simulink model "MyBatteryCU_RTW"  (Simulink 8.7)
settings: Solver=ode1  SolverMode=SingleTasking  StartTime=0.0  StopTime=inf  FixedStep=0.0002  RelTol=1e-3
PreLoadFcn:
  | vehicle = 'Car'; if ~length(which('cmcmd')), cmenv; end
  | MyBatteryCU_RTW_bus
InitFcn:
  | vehicle = 'Car'; if ~length(which('cmcmd')), cmenv; end
  | MyBatteryCU_RTW_bus
Description:
  | CarMaker Plug-in Model Target
settings Model: Creator=ml  LastModifiedBy=IPG
settings DataIOCC: SignalLoggingSaveFormat=ModelDataLogs
settings OptimizationCC: ExpressionDepthLimit=2147483647
settings DebuggingCC: FcnCallInpInsideContextMsg=UseLocalSettings  StateNameClashWarn=warning
settings HardwareCC: TargetHWDeviceType=32-bit Generic  ProdEqTarget=off
settings RTWCC: SystemTargetFile=CarMaker.tlc  TemplateMakefile=CarMaker_unix-win64.tmf  Description=CarMaker Plug-in Model Target
settings CodeAppCC: MaxIdLength=63
settings STFCustomTargetCC: ModelReferenceCompliant=off  GeneratePreprocessorConditionals=Disable all  MultiInstanceERTCode=on  CodeInterfacePackaging=Reusable function  CPPClassGenCompliant=on  GRTInterface=off  GenerateAllocFcn=on  SystemTargetFile=CarMaker.tlc
settings GRTTargetCC: ModelReferenceCompliant=off  ParMdlRefBuildCompliant=off  CompOptLevelCompliant=off  ConcurrentExecutionCompliant=off  CombineOutputUpdateFcns=off  MatFileLogging=off  MultiInstanceERTCode=on  CodeInterfacePackaging=Reusable function  GenerateAllocFcn=on  UseToolchainInfoCompliant=off  ExtModeMexFile=noextcomm
settings CustomProperty: DataType=string  Value=..
settings EnumStrPairs: String=Car

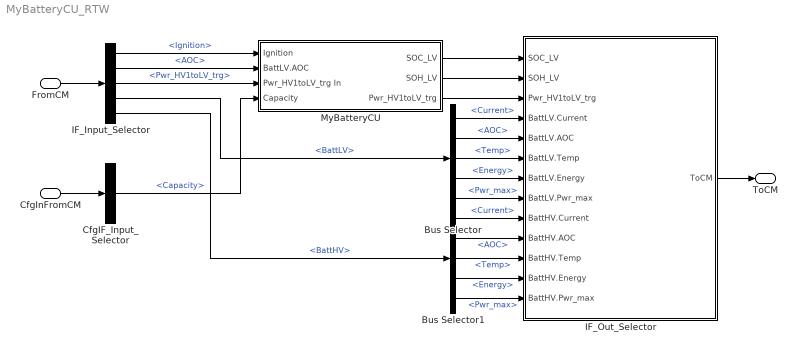
== system MyBatteryCU_RTW ==
  FromCM : Inport  OutDataTypeStr=Bus: cmPTBatteryCUIn
  CfgInFromCM : Inport  Port=2  OutDataTypeStr=Bus: cmPTBatteryCUCfgIn
  Bus Selector : BusSelector  OutputSignals=Current,AOC,Temp,Energy,Pwr_max
  Bus Selector1 : BusSelector  OutputSignals=Current,AOC,Temp,Energy,Pwr_max
  CfgIF_Input_Selector : BusSelector  OutputSignals=BattLV.Capacity
  IF_Input_Selector : BusSelector  OutputSignals=Ignition,BattLV.AOC,Pwr_HV1toLV_trg,BattLV,BattHV
  IF_Out_Selector : Subsystem  mask(Signal Selection){}
      mask help: Signal Selection Block
      settings: OpenFcn=cmSignalSelect('SignalSelection_CB',gcb)
  MyBatteryCU : Subsystem
  ToCM : Outport  OutDataTypeStr=Bus: cmPTBatteryCUOut
  wires:
  FromCM/1 -> IF_Input_Selector/1
  IF_Out_Selector/1(ToCM) -> ToCM/1
  CfgInFromCM/1 -> CfgIF_Input_Selector/1
  MyBatteryCU/1(SOC_LV) -> IF_Out_Selector/1(SOC_LV)
  MyBatteryCU/2(SOH_LV) -> IF_Out_Selector/2(SOH_LV)
  MyBatteryCU/3(Pwr_HV1toLV_trg) -> IF_Out_Selector/3(Pwr_HV1toLV_trg)
  IF_Input_Selector/1 -> MyBatteryCU/1(Ignition)  "<Ignition>"
  CfgIF_Input_Selector/1 -> MyBatteryCU/4(Capacity)  "<Capacity>"
  IF_Input_Selector/2 -> MyBatteryCU/2(BattLV.AOC)  "<AOC>"
  IF_Input_Selector/3 -> MyBatteryCU/3(Pwr_HV1toLV_trg In)  "<Pwr_HV1toLV_trg>"
  IF_Input_Selector/4 -> Bus Selector/1  "<BattLV>"
  IF_Input_Selector/5 -> Bus Selector1/1  "<BattHV>"
  Bus Selector/1 -> IF_Out_Selector/4(BattLV.Current)  "<Current>"
  Bus Selector/2 -> IF_Out_Selector/5(BattLV.AOC)  "<AOC>"
  Bus Selector/3 -> IF_Out_Selector/6(BattLV.Temp)  "<Temp>"
  Bus Selector/4 -> IF_Out_Selector/7(BattLV.Energy)  "<Energy>"
  Bus Selector/5 -> IF_Out_Selector/8(BattLV.Pwr_max)  "<Pwr_max>"
  Bus Selector1/1 -> IF_Out_Selector/9(BattHV.Current)  "<Current>"
  Bus Selector1/2 -> IF_Out_Selector/10(BattHV.AOC)  "<AOC>"
  Bus Selector1/3 -> IF_Out_Selector/11(BattHV.Temp)  "<Temp>"
  Bus Selector1/4 -> IF_Out_Selector/12(BattHV.Energy)  "<Energy>"
  Bus Selector1/5 -> IF_Out_Selector/13(BattHV.Pwr_max)  "<Pwr_max>"

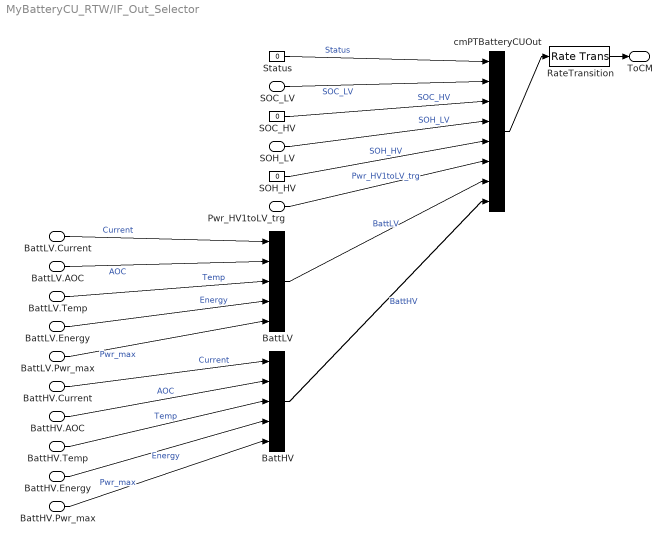
== system MyBatteryCU_RTW/IF_Out_Selector ==
  SOC_LV : Inport
  SOH_LV : Inport  Port=2
  Pwr_HV1toLV_trg : Inport  Port=3
  BattLV.Current : Inport  Port=4
  BattLV.AOC : Inport  Port=5
  BattLV.Temp : Inport  Port=6
  BattLV.Energy : Inport  Port=7
  BattLV.Pwr_max : Inport  Port=8
  BattHV.Current : Inport  Port=9
  BattHV.AOC : Inport  Port=10
  BattHV.Temp : Inport  Port=11
  BattHV.Energy : Inport  Port=12
  BattHV.Pwr_max : Inport  Port=13
  BattHV : BusCreator  Inputs=5
  BattLV : BusCreator  Inputs=5
  RateTransition : RateTransition  OutPortSampleTime=str2num(get_param(bdroot,'FixedStep'))
  SOC_HV : Constant  Value=0
  SOH_HV : Constant  Value=0
  Status : Constant  Value=0
  cmPTBatteryCUOut : BusCreator  Inputs=8
  ToCM : Outport
  wires:
  RateTransition/1 -> ToCM/1
  cmPTBatteryCUOut/1 -> RateTransition/1
  Status/1 -> cmPTBatteryCUOut/1  "Status"
  SOC_HV/1 -> cmPTBatteryCUOut/3  "SOC_HV"
  SOH_HV/1 -> cmPTBatteryCUOut/5  "SOH_HV"
  BattLV/1 -> cmPTBatteryCUOut/7  "BattLV"
  BattHV/1 -> cmPTBatteryCUOut/8  "BattHV"
  SOC_LV/1 -> cmPTBatteryCUOut/2  "SOC_LV"
  SOH_LV/1 -> cmPTBatteryCUOut/4  "SOH_LV"
  Pwr_HV1toLV_trg/1 -> cmPTBatteryCUOut/6  "Pwr_HV1toLV_trg"
  BattLV.Current/1 -> BattLV/1  "Current"
  BattLV.AOC/1 -> BattLV/2  "AOC"
  BattLV.Temp/1 -> BattLV/3  "Temp"
  BattLV.Energy/1 -> BattLV/4  "Energy"
  BattLV.Pwr_max/1 -> BattLV/5  "Pwr_max"
  BattHV.Current/1 -> BattHV/1  "Current"
  BattHV.AOC/1 -> BattHV/2  "AOC"
  BattHV.Temp/1 -> BattHV/3  "Temp"
  BattHV.Energy/1 -> BattHV/4  "Energy"
  BattHV.Pwr_max/1 -> BattHV/5  "Pwr_max"

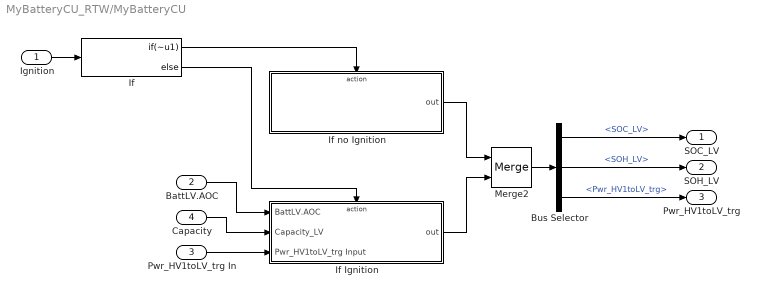
== system MyBatteryCU_RTW/MyBatteryCU ==
  Ignition : Inport
  BattLV.AOC : Inport  Port=2
  Pwr_HV1toLV_trg In : Inport  Port=3
  Capacity : Inport  Port=4
  Bus Selector : BusSelector  OutputSignals=SOC_LV,SOH_LV,Pwr_HV1toLV_trg
  If : If  IfExpression=~u1
  If Ignition : Subsystem  TreatAsAtomicUnit=on
  If no Ignition : Subsystem  TreatAsAtomicUnit=on
  Merge2 : Merge
  SOC_LV : Outport
  SOH_LV : Outport  Port=2
  Pwr_HV1toLV_trg : Outport  Port=3
  wires:
  Ignition/1 -> If/1
  If/1 -> If no Ignition/Action
  BattLV.AOC/1 -> If Ignition/1(BattLV.AOC)
  Capacity/1 -> If Ignition/2(Capacity_LV)
  Pwr_HV1toLV_trg In/1 -> If Ignition/3(Pwr_HV1toLV_trg Input)
  If/2 -> If Ignition/Action
  Merge2/1 -> Bus Selector/1
  If Ignition/1(out) -> Merge2/2
  If no Ignition/1(out) -> Merge2/1
  Bus Selector/1 -> SOC_LV/1  "<SOC_LV>"
  Bus Selector/2 -> SOH_LV/1  "<SOH_LV>"
  Bus Selector/3 -> Pwr_HV1toLV_trg/1  "<Pwr_HV1toLV_trg>"

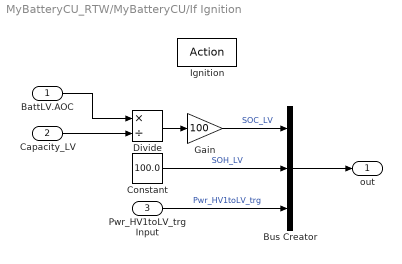
== system MyBatteryCU_RTW/MyBatteryCU/If Ignition ==
  BattLV.AOC : Inport
  Capacity_LV : Inport  Port=2
  Pwr_HV1toLV_trg Input : Inport  Port=3
  Ignition : ActionPort  ActionType=else
  Bus Creator : BusCreator  Inputs=3
  Constant : Constant  Value=100.0
  Divide : Product  Inputs=*/
  Gain : Gain  Gain=100
  out : Outport  InitialOutput=[,100,]
  wires:
  Constant/1 -> Bus Creator/2  "SOH_LV"
  BattLV.AOC/1 -> Divide/1
  Capacity_LV/1 -> Divide/2
  Divide/1 -> Gain/1
  Gain/1 -> Bus Creator/1  "SOC_LV"
  Pwr_HV1toLV_trg Input/1 -> Bus Creator/3  "Pwr_HV1toLV_trg"
  Bus Creator/1 -> out/1

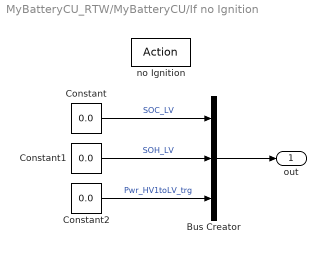
== system MyBatteryCU_RTW/MyBatteryCU/If no Ignition ==
  no Ignition : ActionPort  ActionType=then
  Bus Creator : BusCreator  Inputs=3
  Constant : Constant  Value=0.0
  Constant1 : Constant  Value=0.0
  Constant2 : Constant  Value=0.0
  out : Outport  InitialOutput=0
  wires:
  Constant1/1 -> Bus Creator/2  "SOH_LV"
  Constant/1 -> Bus Creator/1  "SOC_LV"
  Constant2/1 -> Bus Creator/3  "Pwr_HV1toLV_trg"
  Bus Creator/1 -> out/1
